simulink model "Graph_all"  (R2018b)
settings: Solver=FixedStepAuto  StartTime=0.0  StopTime=10.0  FixedStep=0.001  RelTol=1e-3
settings Model: Creator=kekos  LastModifiedBy=kekos

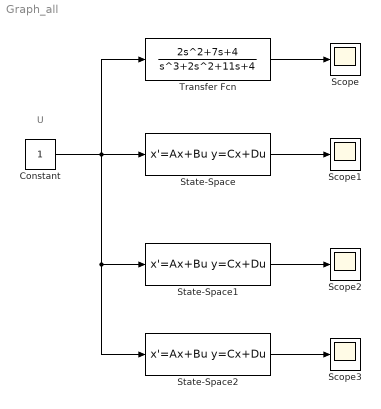
== system Graph_all ==
  note: U
  Constant : Constant
  Scope{,1..3} (4 alike) : Scope
  State-Space : StateSpace  A=[0 1 0; 0 0 1; -4 -11 -2;]  B=[0; 0; 1;]  C=[4 7 2;]  InitialCondition=0
  State-Space1 : StateSpace  A=[0 0 -4; 1 0 -11; 0 1 -2;]  B=[4; 7; 2;]  C=[0 0 1]  InitialCondition=0
  State-Space2 : StateSpace  A=[-0.3854 0 0; 0 -0.8073 3.1187; 0 -3.1187 -0.8073;]  B=[0.1615; -3.926; 2.3114;]  C=[1 1 1]  InitialCondition=0
  Transfer Fcn : TransferFcn  Numerator=[2 7 4]  Denominator=[1 2 11 4]
  wires:
  State-Space1/1 -> Scope2/1
  State-Space/1 -> Scope1/1
  Transfer Fcn/1 -> Scope/1
  Constant/1 -> State-Space2/1, State-Space1/1, Transfer Fcn/1, State-Space/1
  State-Space2/1 -> Scope3/1
